simulink model "Joint_Space_Inv_Dyn"  (R2020b)
settings: Solver=VariableStepAuto  StartTime=0.0  StopTime=2  RelTol=1e-3
values from neighbouring files (symbols this model uses):
  B = myRobot.B_Lagrangian    [hw7_main.m]
  C = myRobot.C_Lagrangian    [hw7_main.m]
  F = myRobot.F    [hw7_main.m]
  G = myRobot.G_Lagrangian    [hw7_main.m]
  Kd = diag([1 1 1]).*0    [hw7_main.m]
  Kp = diag([1 1 1]).*0    [hw7_main.m]
  Ts = 0.001    [hw7_main.m]
settings Model: Creator=nicol  LastModifiedBy=nicol

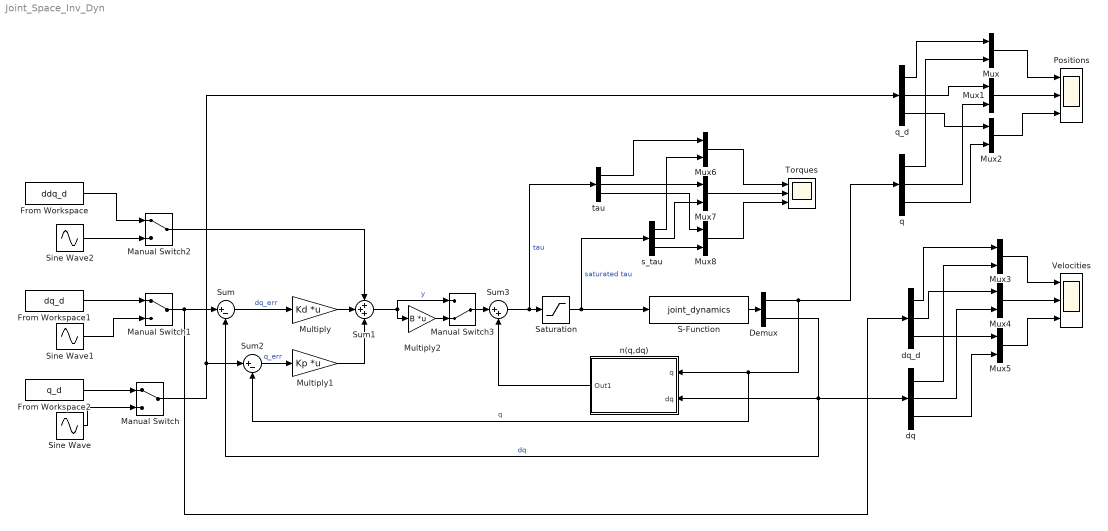
== system Joint_Space_Inv_Dyn ==
  Demux : Demux  Outputs=2
  From Workspace : FromWorkspace  VariableName=ddq_d  SampleTime=Ts
  From Workspace1 : FromWorkspace  VariableName=dq_d  SampleTime=Ts
  From Workspace2 : FromWorkspace  VariableName=q_d  SampleTime=Ts
  Manual Switch : ManualSwitch
  Manual Switch1 : ManualSwitch
  Manual Switch2 : ManualSwitch
  Manual Switch3 : ManualSwitch  CurrentSetting=0
  Multiply : Gain  Gain=Kd  Multiplication=Matrix(K*u)
  Multiply1 : Gain  Gain=Kp  Multiplication=Matrix(K*u)
  Multiply2 : Gain  Gain=B  Multiplication=Matrix(K*u)
  Mux{,1..8} (9 alike) : Mux  Inputs=2
  Positions : Scope  NumInputPorts=3
  S-Function : S-Function  FunctionName=joint_dynamics  Parameters=myRobot  SFunctionDeploymentMode=off  EnableBusSupport=off
  Saturation : Saturate  UpperLimit=50  LowerLimit=-50
  Sine Wave : Sin  Amplitude=0.1  SampleTime=0  VectorParams1D=off
  Sine Wave1 : Sin  Amplitude=0.1  SampleTime=0  VectorParams1D=off
  Sine Wave2 : Sin  Amplitude=0.1  SampleTime=0  VectorParams1D=off
  Sum : Sum  Inputs=|+-
  Sum1 : Sum  Inputs=+++
  Sum2 : Sum  Inputs=|+-
  Sum3 : Sum  Inputs=|++
  Torques : Scope  NumInputPorts=3
  Velocities : Scope  NumInputPorts=3
  dq : Demux  Outputs=3
  dq_d : Demux  Outputs=3
  n(q,dq) : Subsystem
  q : Demux  Outputs=3
  q_d : Demux  Outputs=3
  s_tau : Demux  Outputs=3
  tau : Demux  Outputs=3
  wires:
  From Workspace1/1 -> Manual Switch1/1
  Sum/1 -> Multiply/1  "dq_err"
  Multiply/1 -> Sum1/2
  From Workspace2/1 -> Manual Switch/1
  Sum2/1 -> Multiply1/1  "q_err"
  Multiply1/1 -> Sum1/3
  Multiply2/1 -> Manual Switch3/2
  Sum3/1 -> tau/1, Saturation/1  "tau"
  S-Function/1 -> Demux/1
  Demux/1 -> q/1, n(q,dq)/1(q), Sum2/2  "q"
  Demux/2 -> n(q,dq)/2(dq), Sum/2, dq/1  "dq"
  Sum1/1 -> Multiply2/1, Manual Switch3/1  "y"
  n(q,dq)/1(Out1) -> Sum3/2
  From Workspace/1 -> Manual Switch2/1
  q/2 -> Mux1/2
  q/3 -> Mux2/2
  q/1 -> Mux/2
  Sine Wave/1 -> Manual Switch/2
  Sine Wave1/1 -> Manual Switch1/2
  Sine Wave2/1 -> Manual Switch2/2
  Manual Switch2/1 -> Sum1/1
  Manual Switch1/1 -> dq_d/1, Sum/1
  q_d/1 -> Mux/1
  q_d/2 -> Mux1/1
  q_d/3 -> Mux2/1
  Mux/1 -> Positions/1
  Mux1/1 -> Positions/2
  Mux2/1 -> Positions/3
  Mux3/1 -> Velocities/1
  dq_d/3 -> Mux5/1
  Mux4/1 -> Velocities/2
  Mux5/1 -> Velocities/3
  dq_d/2 -> Mux4/1
  dq/1 -> Mux3/2
  dq_d/1 -> Mux3/1
  dq/3 -> Mux5/2
  Manual Switch/1 -> q_d/1, Sum2/1
  dq/2 -> Mux4/2
  Saturation/1 -> S-Function/1, s_tau/1  "saturated tau"
  tau/2 -> Mux7/1
  tau/1 -> Mux6/1
  s_tau/1 -> Mux6/2
  s_tau/2 -> Mux7/2
  tau/3 -> Mux8/1
  s_tau/3 -> Mux8/2
  Mux6/1 -> Torques/1
  Mux7/1 -> Torques/2
  Mux8/1 -> Torques/3
  Manual Switch3/1 -> Sum3/1

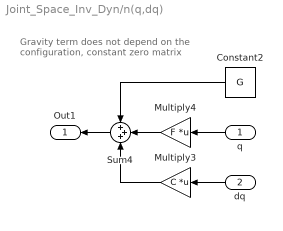
== system Joint_Space_Inv_Dyn/n(q,dq) ==
  note: Gravity term does not depend on the
      |  configuration, constant zero matrix
  q : Inport
  dq : Inport  Port=2
  Constant2 : Constant  Value=G  VectorParams1D=off
  Multiply3 : Gain  Gain=C  Multiplication=Matrix(K*u)
  Multiply4 : Gain  Gain=F  Multiplication=Matrix(K*u)
  Sum4 : Sum  Inputs=+++
  Out1 : Outport
  wires:
  Sum4/1 -> Out1/1
  Multiply3/1 -> Sum4/3
  Multiply4/1 -> Sum4/2
  Constant2/1 -> Sum4/1
  q/1 -> Multiply4/1
  dq/1 -> Multiply3/1
